simulink model "Reaching"  (R2024a)
settings: Solver=ode23t  StartTime=0.0  StopTime=inf  FixedStep=0.001  RelTol=1e-3
undefined symbols (not defined in the file): get
libraries: vrlib x2, PhanTorque_3Dof_Library_64Bits x1
settings Model: Creator=carlos.aldana  LastModifiedBy=amisq
settings SolverCC: AlgebraicLoopSolver=TrustRegion
settings DataIOCC: LimitDataPoints=on  SaveFormat=Array  ReturnWorkspaceOutputs=off
settings OptimizationCC: BlockReduction=off  BooleanDataType=off  LifeSpan=inf
settings DebuggingCC: SaveWithParameterizedLinksMsg=none  UnderspecifiedInitializationDetection=Classic  MergeDetectMultiDrivingBlocksExec=none  SignalResolutionControl=TryResolveAllWithWarning  UnconnectedInputMsg=warning  UnconnectedOutputMsg=warning  UnconnectedLineMsg=warning  AllowSymbolicDim=off  SFUnexpectedBacktrackingDiag=warning  SFNoUnconditionalDefaultTransitionDiag=warning  SFExecutionAtInitializationDiag=none  ArithmeticOperatorsInVariantConditions=warning
settings HardwareCC: ProdBitPerPointer=32  ProdBitPerSizeT=32  ProdBitPerPtrDiffT=32  ProdLargestAtomicFloat=None  ProdIntDivRoundTo=Undefined  ProdEndianess=Unspecified  ProdWordSize=32  ProdHWDeviceType=32-bit Generic  TargetUnknown=on
settings ModelReferenceCC: EnableRefExpFcnMdlSchedulingChecks=on  PropagateSignalLabelsOutOfModel=off
settings SFSimCC: SimUseLocalCustomCode=off  CustomCodeUndefinedFunction=UseInterfaceOnly
settings RTWCC: RTWUseLocalCustomCode=off  GPUComputeCapability=3.5  DLArmComputeVersion=19.05
settings CodeAppCC: StateflowObjectComments=on
settings GRTTargetCC: TargetLangStandard=C89/C90 (ANSI)
settings ConfigComp: CovMetricSettings=dw  CovSaveCumulativeToWorkspaceVar=on  CovSaveSingleToWorkspaceVar=on  CovExternalEMLEnable=off  CovSFcnEnable=off

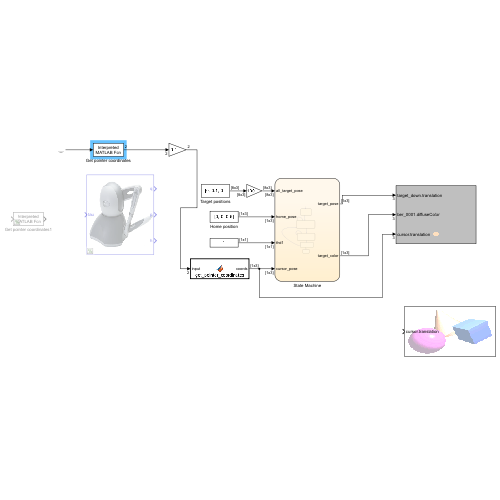
[thumbnail: Simulink's stored preview of the top-level diagram]
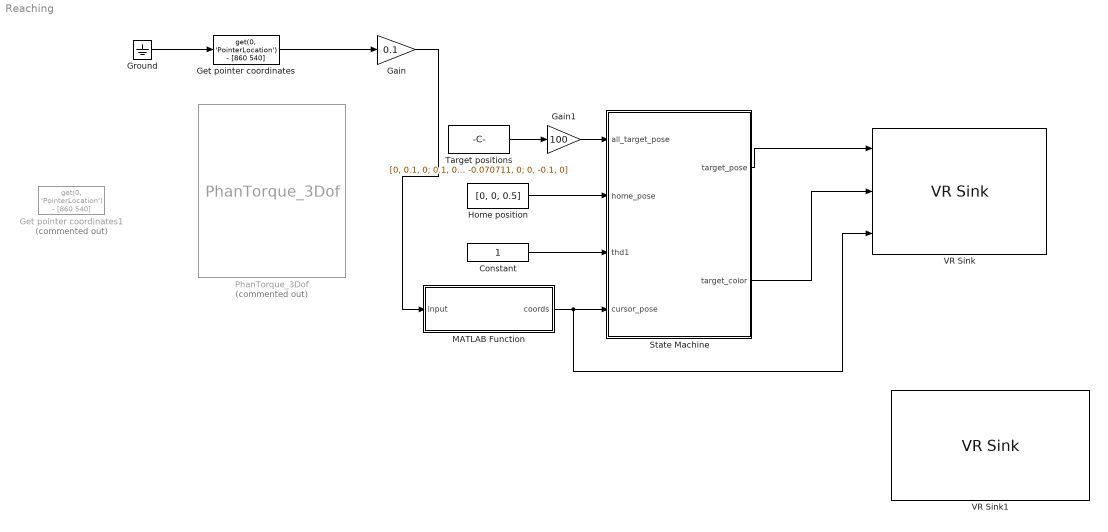
== system Reaching ==
  Constant : Constant  VectorParams1D=off
  Gain : Gain  Gain=0.1
  Gain1 : Gain  Gain=100
  Get pointer coordinates : MATLABFcn  MATLABFcn=get(0, 'PointerLocation') - [860 540]  OutputDimensions=2
  Get pointer coordinates1 : MATLABFcn  Commented=on  MATLABFcn=get(0, 'PointerLocation') - [860 540]  OutputDimensions=2
  Ground : Ground
  Home position : Constant  Value=[0, 0, 0.5]  VectorParams1D=off
  MATLAB Function : MATLAB Function  TreatAsAtomicUnit=on
  PhanTorque_3Dof : PhanTorque_3Dof_Library_64Bits/PhanTorque_3Dof  Commented=on  Haptic_Name='Default Device'
  State Machine : Stateflow chart  TreatAsAtomicUnit=on
  Target positions : Constant  Value=[0, 0.1, 0; 0.1, 0, 0; -0.1, 0, 0; 0.070711, 0.070711, 0; -0.070711, -0.070711, 0; -0.070711, 0.070711, 0; 0.070711, -0.070711, 0; 0, -0.1, 0]  VectorParams1D=off
  VR Sink : vrlib/VR Sink  InstantiateOnLoad=on  SampleTime=0.1  ViewEnable=on  RemoteChange=off  RemoteView=off  FieldsWritten=target_down.translation.3.1.1.double#ber_0001.diffuseColor.3.1.1.double#cursor.translation.3.1.1.double  WorldFileName=VR_centerAndTarget.wrl  AutoView=off  VideoDimensions=[]  AllowVariableSize=off  FigureProperties="{'Position', 'Name', 'Viewpoint', 'CameraBound', 'CameraDirection', 'CameraPosition', 'CameraUpVector', 'ZoomFactor', 'Antialiasing', 'Headlight', 'Lighting', 'Sound', 'StatusBar', 'Stereo3D', 'Stereo3DCameraOffset', 'Stereo3DHIT', 'ToolBar', 'Textures', 'Transparency', 'Triad', 'Wireframe', 'NavZones', 'NavMode', 'NavSpeed', 'CaptureFileFormat', 'CaptureFileName', 'Record2DCompressMethod', 'Record2DCompressQuality', 'Record2D', 'Record2DFileName', 'Record2DFPS', 'NavPanel'; [5.0000000000000000e+00   9.2000000000000000e+01   5.7600000000000000e+02   3.5000000000000000e+02], '', '_untitled_1', 'on', [0.0000000000000000e+00   0.0000000000000000e+00  -1.0000000000000000e+00], [0.0000000000000000e+00   0.0000000000000000e+00   0.0000000000000000e+00], [0.0000000000000000e+00   1.0000000000000000e+00   0.0000000000000000e+00], [1.0000000000000000e+00], 'on', 'on', 'on', 'on', 'on', 'off', [1.0000000149011612e-01], [0.0000000000000000e+00], 'on', 'on', 'on', 'none', 'off', 'off', 'fly', 'normal', 'tif', '%f_anim_%n.tif', 'auto', [7.5000000000000000e+01], 'off', '%f_anim_%n.avi', 'auto', 'halfbar'}"
  VR Sink1 : vrlib/VR Sink  InstantiateOnLoad=on  SampleTime=0.1  ViewEnable=on  RemoteChange=off  RemoteView=off  FieldsWritten=cursor.translation.3.1.1.double  WorldFileName=8_palline_color.wrl  AutoView=off  VideoDimensions=[]  AllowVariableSize=off
  wires:
  Get pointer coordinates/1 -> Gain/1
  Ground/1 -> Get pointer coordinates/1
  Target positions/1 -> Gain1/1
  Home position/1 -> State Machine/2(home_pose)
  Constant/1 -> State Machine/3(thd1)
  State Machine/1(target_pose) -> VR Sink/1
  State Machine/2(target_color) -> VR Sink/2
  MATLAB Function/1(coords) -> VR Sink/3, State Machine/4(cursor_pose)
  Gain/1 -> MATLAB Function/1(input)
  Gain1/1 -> State Machine/1(all_target_pose)

== stateflow chart Reaching/State Machine ==
  state Initializing
    entry:
    counter = 1
    target_color = [1 0 0]
    target_pose = zeros(1,3)
    target_pose = home_pose
  state reach_target
    entry:
    target_color = [0 1 0]
    target_pose = all_target_pose(counter, :)
  state reach_home
    entry:
    target_color = [1 0 0]
    target_pose = home_pose
  state increase_counter
    entry:
    counter = counter + 1
  state Finish
  (default) -> Initializing
  Initializing -> reach_target : [norm(cursor_pose(1:2) - home_pose(1:2)) <= thd1]
  reach_target -> reach_target [order 2] : [norm(cursor_pose(1:2) - target_pose(1:2)) > thd1]
  increase_counter -> reach_target [order 2]
  reach_target -> reach_home [order 1] : [norm(cursor_pose(1:2) - target_pose(1:2)) <= thd1 && after(1, sec)]
  reach_home -> reach_home [order 1] : [norm(cursor_pose(1:2) - home_pose(1:2)) > thd1]
  reach_home -> increase_counter [order 2] : [norm(cursor_pose(1:2) - home_pose(1:2)) <= thd1 && after(2, sec)]
  increase_counter -> Finish [order 1] : [counter == 9]
  data: target_pose output; all_target_pose input; home_pose input; thd1 input; cursor_pose input; counter local; time local; radius local; angle local; target_color output; thd constant double

== matlab function Reaching/MATLAB Function ==
  data: coords output; input input
function coords = get_pointer_coordinates(input)  
    coords = [input(1), input(2), 1.5]; 
end
